simulink model "agent_test_ST_impl"  (R2015a)
settings: Solver=ode1  StartTime=0.0  StopTime=Inf  FixedStep=0.1  RelTol=1e-3
model workspace (MAT data in the model file):
  SL_ROS_VariableLengthArrays_MaxSizes.CommonInfo.ArrayTruncateAction = 'EmitWarning'
  SL_ROS_VariableLengthArrays_MaxSizes.MsgTypeMap = containers.Map
  SL_ROS_VariableLengthArrays_MaxSizes.MsgTypeMap.serialization.keys = {'agent_test/FormationStatisticsArray'}
  SL_ROS_VariableLengthArrays_MaxSizes.MsgTypeMap.serialization.values{1}(1).PropertyName = 'Neighbours'
  SL_ROS_VariableLengthArrays_MaxSizes.MsgTypeMap.serialization.values{1}(1).DataType = 'int32'
  SL_ROS_VariableLengthArrays_MaxSizes.MsgTypeMap.serialization.values{1}(1).MaxLength = 9
  SL_ROS_VariableLengthArrays_MaxSizes.MsgTypeMap.serialization.values{1}(2).PropertyName = 'Vector'
  SL_ROS_VariableLengthArrays_MaxSizes.MsgTypeMap.serialization.values{1}(2).DataType = 'agent_test/FormationStatisticsStamped'
  SL_ROS_VariableLengthArrays_MaxSizes.MsgTypeMap.serialization.values{1}(2).MaxLength = 9
  SL_ROS_VariableLengthArrays_MaxSizes.MsgTypeMap.serialization.uniformity = 0
  SL_ROS_VariableLengthArrays_MaxSizes.MsgTypeMap.serialization.keyType = 'char'
  SL_ROS_VariableLengthArrays_MaxSizes.MsgTypeMap.serialization.valueType = 'any'
undefined symbols (not defined in the file): k_i_speed
libraries: simulink x2
settings Model: Creator=alextoind  LastModifiedBy=alextoind

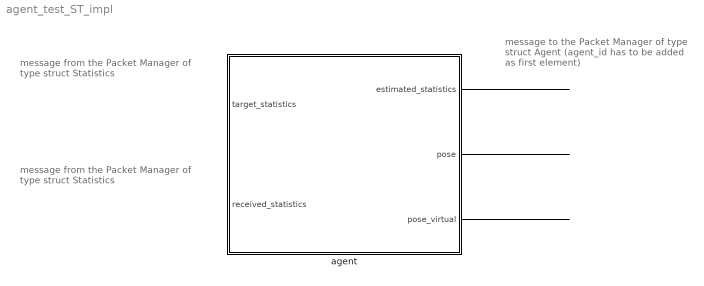
== system agent_test_ST_impl ==
  note: message from the Packet Manager of type struct Statistics
  note: message from the Packet Manager of type struct Statistics
  note: message to the Packet Manager of type struct Agent (agent_id has to be added as first element)
  agent : Subsystem  InitFcn=|  mask{agent_id=1, pose_0=[-0.5, -0.5, 0], pose_virtual_0=[-0.5, -0.5, 0], gamma=diag([100, 100, 5, 10, 5]), lambda=diag([0, 0, 0, 0, 0]), B=diag([100, 100]), k_p_speed=0.5, k_p_steer=2.0, vehicle_length=0.4, speed_min=0.0, speed_max=4.0, steer_min=-0.25, steer_max=0.25, velocity_virtual_threshold=4.0}
      | rosshutdown;
      | robotics.ros.createSimulinkBus(gcs);
      | rosinit;
      | 
      | vehicle_length = 0.4;
      | 
      | velocity_virtual_threshold = 2.0;
      | los_distance_threshold = 4.0;
      | 
      | speed_min = 0.0;
      | speed_max = 4.0;
      | steer_min =  -0.52;
      | steer_max = 0.52;
      | 
      | k_p_speed = 0.5;
      | k_i_speed = 0.0;
      | k_p_steer = 1.5;
      | 
      | gamma = diag([100, 100, 5, 10, 5]);
      | lambda = diag([0, 0, 0, 0, 0]);
      | B = diag([100, 100]);
      mask prompts: agent_id "Agent ID (choose a number from 1 to 9)"; pose_0 "Initial Agent Pose (x, y, theta)"; pose_virtual_0 "Initial Virtual Agent Pose (x, y, theta)"; gamma "Gamma Matrix (5x5)"; lambda "Lambda Matrix (5x5)"; B "B Matrix (2x2)"; k_p_speed "Speed Proportional Gain"; k_p_steer "Steer Proportional Gain"; vehicle_length "Vehicle Length (m)"; speed_min "Speed Lower Bound (m/s)"; speed_max "Speed Upper Bound (m/s)"; steer_min "Steer Lower Bound (rad/s)"; steer_max "Steer Upper Bound (rad/s)"; velocity_virtual_threshold "Speed Virtual Threshold (m/s)"
  wires:
  ? -> agent/1(target_statistics)
  ? -> agent/2(received_statistics)
  agent/1(estimated_statistics) -> ?
  agent/2(pose) -> ?
  agent/3(pose_virtual) -> ?

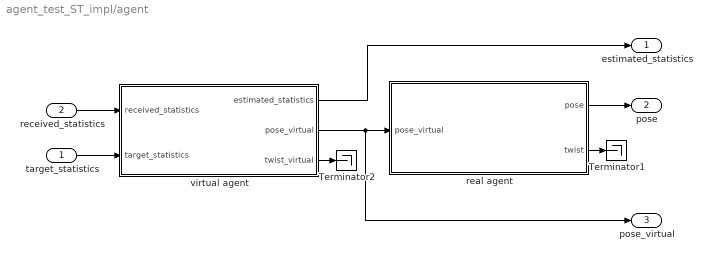
== system agent_test_ST_impl/agent ==
  target_statistics : Inport
  received_statistics : Inport  Port=2
  Terminator1 : Terminator
  Terminator2 : Terminator
  real agent : Subsystem  TreatAsAtomicUnit=on
  virtual agent : Subsystem  TreatAsAtomicUnit=on
  estimated_statistics : Outport
  pose : Outport  Port=2
  pose_virtual : Outport  Port=3
  wires:
  virtual agent/2(pose_virtual) -> pose_virtual/1, real agent/1(pose_virtual)
  virtual agent/1(estimated_statistics) -> estimated_statistics/1
  real agent/2(twist) -> Terminator1/1
  virtual agent/3(twist_virtual) -> Terminator2/1
  real agent/1(pose) -> pose/1
  received_statistics/1 -> virtual agent/1(received_statistics)
  target_statistics/1 -> virtual agent/2(target_statistics)

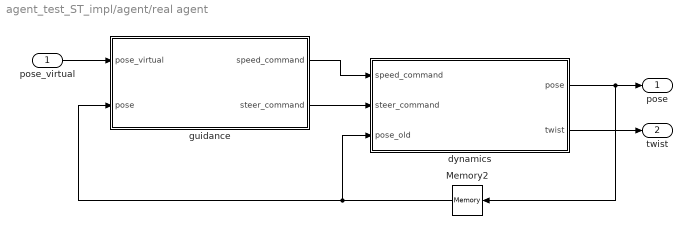
== system agent_test_ST_impl/agent/real agent ==
  pose_virtual : Inport
  Memory2 : Memory  X0=pose_0
  dynamics : Subsystem
  guidance : Subsystem
  pose : Outport
  twist : Outport  Port=2
  wires:
  pose_virtual/1 -> guidance/1(pose_virtual)
  guidance/1(speed_command) -> dynamics/1(speed_command)
  guidance/2(steer_command) -> dynamics/2(steer_command)
  dynamics/1(pose) -> Memory2/1, pose/1
  dynamics/2(twist) -> twist/1
  Memory2/1 -> guidance/2(pose), dynamics/3(pose_old)

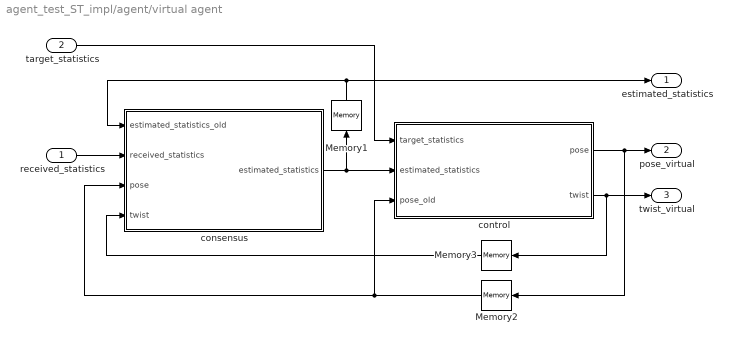
== system agent_test_ST_impl/agent/virtual agent ==
  received_statistics : Inport
  target_statistics : Inport  Port=2
  Memory1 : Memory  X0=[0, 0, 0, 0, 0]
  Memory2 : Memory  X0=pose_virtual_0
  Memory3 : Memory  X0=[0;0;0]
  consensus : Subsystem
  control : Subsystem
  estimated_statistics : Outport
  pose_virtual : Outport  Port=2
  twist_virtual : Outport  Port=3
  wires:
  received_statistics/1 -> consensus/2(received_statistics)
  target_statistics/1 -> control/1(target_statistics)
  control/1(pose) -> Memory2/1, pose_virtual/1
  control/2(twist) -> Memory3/1, twist_virtual/1
  consensus/1(estimated_statistics) -> control/2(estimated_statistics), Memory1/1
  Memory2/1 -> control/3(pose_old), consensus/3(pose)
  Memory1/1 -> estimated_statistics/1, consensus/1(estimated_statistics_old)
  Memory3/1 -> consensus/4(twist)

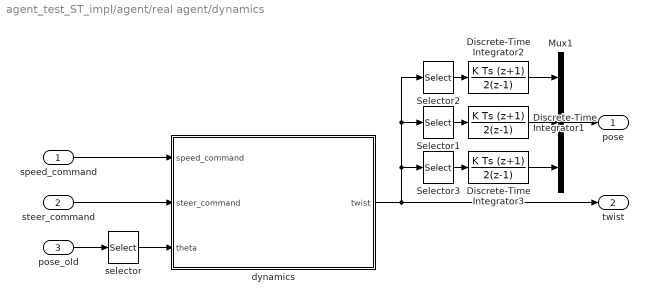
== system agent_test_ST_impl/agent/real agent/dynamics ==
  speed_command : Inport
  steer_command : Inport  Port=2
  pose_old : Inport  Port=3
  Discrete-Time Integrator1 : DiscreteIntegrator  IntegratorMethod=Integration: Trapezoidal  InitialCondition=pose_0(2)  InitialConditionSetting=State (most efficient)  SampleTime=-1
  Discrete-Time Integrator2 : DiscreteIntegrator  IntegratorMethod=Integration: Trapezoidal  InitialCondition=pose_0(1)  InitialConditionSetting=State (most efficient)  SampleTime=-1
  Discrete-Time Integrator3 : DiscreteIntegrator  IntegratorMethod=Integration: Trapezoidal  InitialCondition=pose_0(3)  InitialConditionSetting=State (most efficient)  SampleTime=-1
  Mux1 : Mux  Inputs=3
  Selector1 : Selector  InputPortWidth=3  Indices=[2]
  Selector2 : Selector  InputPortWidth=3  Indices=[1]
  Selector3 : Selector  InputPortWidth=3  Indices=[3]
  dynamics : MATLAB Function  TreatAsAtomicUnit=on
  selector : Selector  InputPortWidth=3  Indices=[3]
  pose : Outport
  twist : Outport  Port=2
  wires:
  steer_command/1 -> dynamics/2(steer_command)
  speed_command/1 -> dynamics/1(speed_command)
  selector/1 -> dynamics/3(theta)
  pose_old/1 -> selector/1
  dynamics/1(twist) -> Selector3/1, Selector1/1, Selector2/1, twist/1
  Discrete-Time Integrator1/1 -> Mux1/2
  Mux1/1 -> pose/1
  Discrete-Time Integrator2/1 -> Mux1/1
  Selector1/1 -> Discrete-Time Integrator1/1
  Selector2/1 -> Discrete-Time Integrator2/1
  Selector3/1 -> Discrete-Time Integrator3/1
  Discrete-Time Integrator3/1 -> Mux1/3

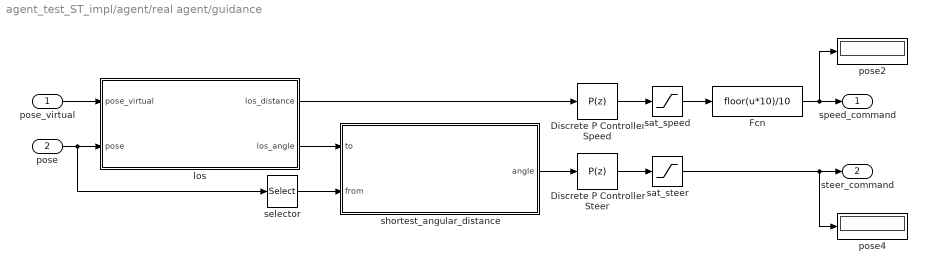
== system agent_test_ST_impl/agent/real agent/guidance ==
  pose_virtual : Inport
  pose : Inport  Port=2
  Discrete P Controller Speed : simulink/Continuous/PID Controller  Controller=P  TimeDomain=Discrete-time  SampleTime=-1  IntegratorMethod=Trapezoidal  FilterMethod=Forward Euler  Form=Parallel  UseFilter=on  ControllerParametersSource=internal  P=k_p_speed  I=k_i_speed  D=0  N=100  InitialConditionSource=internal  InitialConditionForIntegrator=0  InitialConditionForFilter=0  ExternalReset=none  LimitOutput=off  UpperSaturationLimit=inf  LowerSaturationLimit=-inf  LinearizeAsGain=off  AntiWindupMode=none  Kb=1  TrackingMode=off  Kt=1  PParamMin=[]  PParamMax=[]  IParamMin=[]  IParamMax=[]  DParamMin=[]  DParamMax=[]  NParamMin=[]  NParamMax=[]  KbParamMin=[]  KbParamMax=[]  KtParamMin=[]  KtParamMax=[]  POutMin=[]  POutMax=[]  IOutMin=[]  IOutMax=[]  DOutMin=[]  DOutMax=[]  NOutMin=[]  NOutMax=[]  KbOutMin=[]  KbOutMax=[]  KtOutMin=[]  KtOutMax=[]  IntegratorOutMin=[]  IntegratorOutMax=[]  FilterOutMin=[]  FilterOutMax=[]  SumOutMin=[]  SumOutMax=[]  SumI1OutMin=[]  SumI1OutMax=[]  SumI2OutMin=[]  SumI2OutMax=[]  SumI3OutMin=[]  SumI3OutMax=[]  SumDOutMin=[]  SumDOutMax=[]  SaturationOutMin=[]  SaturationOutMax=[]  IntegratorContinuousStateAttributes=''  IntegratorStateMustResolveToSignalObject=off  IntegratorRTWStateStorageClass=Auto  FilterContinuousStateAttributes=''  FilterStateMustResolveToSignalObject=off  FilterRTWStateStorageClass=Auto  DifferentiatorICPrevScaledInput=0  DifferentiatorOutMin=[]  DifferentiatorOutMax=[]
  Discrete P Controller Steer : simulink/Continuous/PID Controller  Controller=P  TimeDomain=Discrete-time  SampleTime=-1  IntegratorMethod=Trapezoidal  FilterMethod=Forward Euler  Form=Parallel  UseFilter=on  ControllerParametersSource=internal  P=k_p_steer  I=k_i_speed  D=0  N=100  InitialConditionSource=internal  InitialConditionForIntegrator=0  InitialConditionForFilter=0  ExternalReset=none  LimitOutput=off  UpperSaturationLimit=inf  LowerSaturationLimit=-inf  LinearizeAsGain=off  AntiWindupMode=none  Kb=1  TrackingMode=off  Kt=1  PParamMin=[]  PParamMax=[]  IParamMin=[]  IParamMax=[]  DParamMin=[]  DParamMax=[]  NParamMin=[]  NParamMax=[]  KbParamMin=[]  KbParamMax=[]  KtParamMin=[]  KtParamMax=[]  POutMin=[]  POutMax=[]  IOutMin=[]  IOutMax=[]  DOutMin=[]  DOutMax=[]  NOutMin=[]  NOutMax=[]  KbOutMin=[]  KbOutMax=[]  KtOutMin=[]  KtOutMax=[]  IntegratorOutMin=[]  IntegratorOutMax=[]  FilterOutMin=[]  FilterOutMax=[]  SumOutMin=[]  SumOutMax=[]  SumI1OutMin=[]  SumI1OutMax=[]  SumI2OutMin=[]  SumI2OutMax=[]  SumI3OutMin=[]  SumI3OutMax=[]  SumDOutMin=[]  SumDOutMax=[]  SaturationOutMin=[]  SaturationOutMax=[]  IntegratorContinuousStateAttributes=''  IntegratorStateMustResolveToSignalObject=off  IntegratorRTWStateStorageClass=Auto  FilterContinuousStateAttributes=''  FilterStateMustResolveToSignalObject=off  FilterRTWStateStorageClass=Auto  DifferentiatorICPrevScaledInput=0  DifferentiatorOutMin=[]  DifferentiatorOutMax=[]
  Fcn : Fcn  Expr=floor(u*10)/10
  los : MATLAB Function  TreatAsAtomicUnit=on
  pose2 : Display
  pose4 : Display
  sat_speed : Saturate  UpperLimit=speed_max  LowerLimit=speed_min
  sat_steer : Saturate  UpperLimit=steer_max  LowerLimit=steer_min
  selector : Selector  InputPortWidth=3  Indices=[3]
  shortest_angular_distance : MATLAB Function  TreatAsAtomicUnit=on
  speed_command : Outport
  steer_command : Outport  Port=2
  wires:
  pose_virtual/1 -> los/1(pose_virtual)
  pose/1 -> los/2(pose), selector/1
  los/2(los_angle) -> shortest_angular_distance/1(to)
  selector/1 -> shortest_angular_distance/2(from)
  shortest_angular_distance/1(angle) -> Discrete P Controller Steer/1
  Discrete P Controller Steer/1 -> sat_steer/1
  Discrete P Controller Speed/1 -> sat_speed/1
  los/1(los_distance) -> Discrete P Controller Speed/1
  sat_speed/1 -> Fcn/1
  Fcn/1 -> pose2/1, speed_command/1
  sat_steer/1 -> pose4/1, steer_command/1

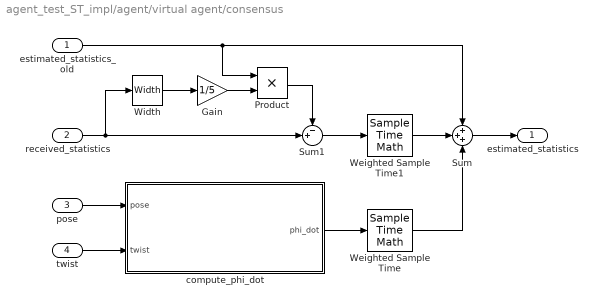
== system agent_test_ST_impl/agent/virtual agent/consensus ==
  estimated_statistics_old : Inport
  received_statistics : Inport  Port=2
  pose : Inport  Port=3
  twist : Inport  Port=4
  Gain : Gain  Gain=1/5
  Product : Product
  Sum : Sum  Inputs=3
  Sum1 : Sum  Inputs=-+|
  Weighted Sample Time : SampleTimeMath  TsampMathOp=*
  Weighted Sample Time1 : SampleTimeMath  TsampMathOp=*
  Width : Width  OutDataTypeMode=All ports same datatype
  compute_phi_dot : MATLAB Function  TreatAsAtomicUnit=on
  estimated_statistics : Outport
  wires:
  pose/1 -> compute_phi_dot/1(pose)
  twist/1 -> compute_phi_dot/2(twist)
  compute_phi_dot/1(phi_dot) -> Weighted Sample Time/1
  estimated_statistics_old/1 -> Product/1, Sum/1
  Weighted Sample Time/1 -> Sum/3
  Sum/1 -> estimated_statistics/1
  Weighted Sample Time1/1 -> Sum/2
  Product/1 -> Sum1/1
  Sum1/1 -> Weighted Sample Time1/1
  received_statistics/1 -> Width/1, Sum1/2
  Width/1 -> Gain/1
  Gain/1 -> Product/2

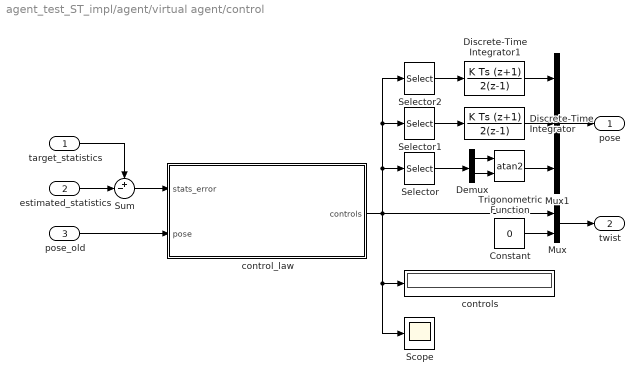
== system agent_test_ST_impl/agent/virtual agent/control ==
  target_statistics : Inport
  estimated_statistics : Inport  Port=2
  pose_old : Inport  Port=3
  Constant : Constant  Value=0
  Demux : Demux  Outputs=2
  Discrete-Time Integrator : DiscreteIntegrator  IntegratorMethod=Integration: Trapezoidal  InitialCondition=pose_virtual_0(2)  InitialConditionSetting=State (most efficient)  SampleTime=-1
  Discrete-Time Integrator1 : DiscreteIntegrator  IntegratorMethod=Integration: Trapezoidal  InitialCondition=pose_virtual_0(1)  InitialConditionSetting=State (most efficient)  SampleTime=-1
  Mux : Mux  Inputs=2
  Mux1 : Mux  Inputs=3
  Scope : Scope
      settings: TimeRange=100  YMin=-0.065  YMax=0  SampleInput=on
  Selector : Selector  InputPortWidth=2  Indices=[2 1]
  Selector1 : Selector  InputPortWidth=2  Indices=[2]
  Selector2 : Selector  InputPortWidth=2  Indices=[1]
  Sum : Sum  Inputs=+-|
  Trigonometric Function : Trigonometry  Operator=atan2
  control_law : MATLAB Function  TreatAsAtomicUnit=on
  controls : Display
  pose : Outport
  twist : Outport  Port=2
  wires:
  pose_old/1 -> control_law/2(pose)
  estimated_statistics/1 -> Sum/2
  target_statistics/1 -> Sum/1
  Sum/1 -> control_law/1(stats_error)
  control_law/1(controls) -> Scope/1, controls/1, Selector1/1, Selector2/1, Selector/1, Mux/1
  Constant/1 -> Mux/2
  Mux/1 -> twist/1
  Discrete-Time Integrator/1 -> Mux1/2
  Mux1/1 -> pose/1
  Trigonometric Function/1 -> Mux1/3
  Selector/1 -> Demux/1
  Demux/2 -> Trigonometric Function/2
  Demux/1 -> Trigonometric Function/1
  Discrete-Time Integrator1/1 -> Mux1/1
  Selector1/1 -> Discrete-Time Integrator/1
  Selector2/1 -> Discrete-Time Integrator1/1

== matlab function agent_test_ST_impl/agent/real agent/dynamics/dynamics ==
  data: speed_command input; steer_command input; twist output; theta input; vehicle_length parameter
function twist = dynamics(speed_command, steer_command, theta, vehicle_length)
%#codegen

  % twist is 2 dimensional (x_dot, y_dot, theta_dot)
  twist = [speed_command * cos(theta); ...
           speed_command * sin(theta); ...
           speed_command * tan(steer_command) / vehicle_length];
end

== matlab function agent_test_ST_impl/agent/virtual agent/consensus/compute_phi_dot ==
  data: pose input; phi_dot output; twist input
function phi_dot = compute_phi_dot(pose, twist)
%#codegen

  phi_dot = [twist(1), ...
             twist(2), ...
             2*pose(1)*twist(1), ...
             pose(2)*twist(1) + pose(1)*twist(2), ...
             2*pose(2)*twist(2)];
end

== matlab function agent_test_ST_impl/agent/virtual agent/control/control_law ==
  data: stats_error input size=[1, 5]; pose input; controls output; B parameter; lambda parameter; gamma parameter; velocity_virtual_threshold parameter
function controls = control_law(stats_error, pose, B, lambda, gamma, velocity_virtual_threshold)
%#codegen

  % jacobian of phi = [px, py, pxx, pxy, pyy]
  J_phi = [eye(2); ...
           2*pose(1), 0; ...
           pose(2),   pose(1); ...
           0,         2*pose(2)];

  controls = (B + J_phi'*lambda*J_phi) \ J_phi'*gamma*stats_error';
  
  % controls saturation
  current_velocity_virtual = norm(controls);
  if current_velocity_virtual > velocity_virtual_threshold
    controls = controls * velocity_virtual_threshold / current_velocity_virtual;
  end
end

== matlab function agent_test_ST_impl/agent/real agent/guidance/los ==
  data: pose_virtual input; pose input; los_distance output; los_angle output
function [los_distance, los_angle] = los(pose_virtual, pose)
%#codegen

  pose_error = pose_virtual - pose;
  los_distance = norm(pose_error(1:2));
  los_angle = atan2(pose_error(2), pose_error(1));
end

== matlab function agent_test_ST_impl/agent/real agent/guidance/shortest_angular_distance ==
  data: to input; from input; angle output
function angle = shortest_angular_distance(to, from)
%#codegen

  angle = normalize_angle_positive(normalize_angle_positive(to) ...
                                   - normalize_angle_positive(from));
  if (angle > pi)
    angle = -(2*pi - angle);
  end
  angle = normalize_angle(angle);
end

function angle_norm = normalize_angle_positive(angle)
  angle_norm = rem(rem(angle, 2*pi) + 2*pi, 2*pi);
end

function angle_norm = normalize_angle(angle)
  angle_norm = normalize_angle_positive(angle);
  if (angle_norm > pi)
    angle_norm = angle_norm - 2*pi;
  end
end
